simulink model "System_Model_Updated_2"  (R2021a)
settings: Solver=VariableStepAuto  StartTime=0.0  StopTime=50  RelTol=1e-3
libraries: pid_lib x4, vrlib x1, sharedutil x1, sharedtransform x1
settings Model: Creator=Hameed  LastModifiedBy=Hameed

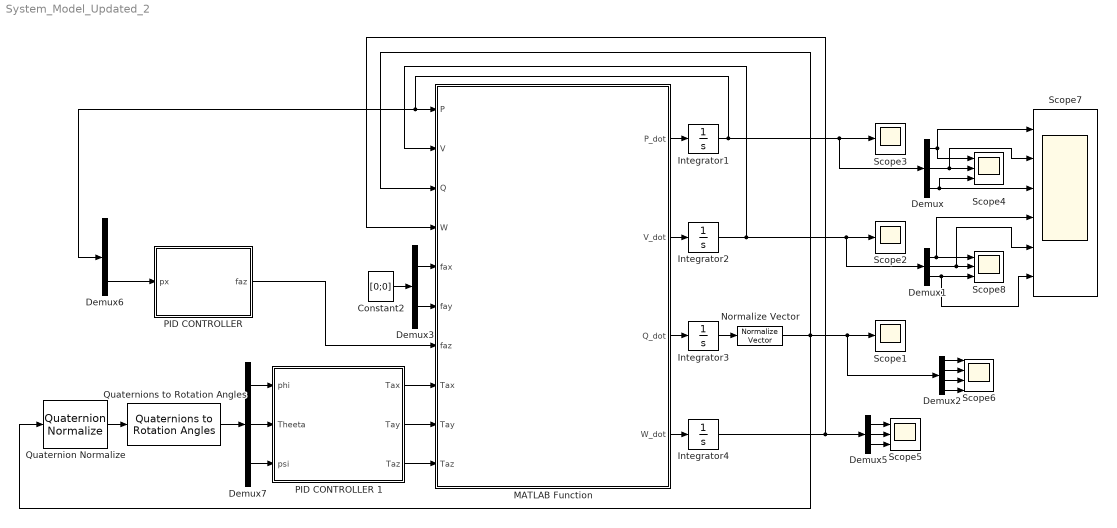
== system System_Model_Updated_2 ==
  Constant2 : Constant  Value=[0;0]  VectorParams1D=off
  Demux{,1,5..7} (5 alike) : Demux  Outputs=3
  Demux2 : Demux
  Demux3 : Demux  Outputs=2
  Integrator1 : Integrator  InitialCondition=[0;0;0]
  Integrator2 : Integrator  InitialCondition=[0;0;0]
  Integrator3 : Integrator  InitialCondition=[1;0;0;0]
  Integrator4 : Integrator  InitialCondition=[0;0;0]
  MATLAB Function : MATLAB Function  TreatAsAtomicUnit=on
  Normalize Vector : vrlib/Utilities/Normalize Vector  maxzero=0
  "PID CONTROLLER " : Subsystem
  PID CONTROLLER 1 : Subsystem
  Quaternion Normalize : sharedutil/Quaternion Normalize  aMode=aMode
      settings: SourceProductBaseCode=AE,PW,DR,MT,UV,VE
  Quaternions to Rotation Angles : sharedtransform/Quaternions to Rotation Angles  rotationOrder=ZYX  aMode=aMode
      settings: SourceProductBaseCode=AE,PW,DR,MT,UV,VE
  Scope1 : Scope
  Scope2 : Scope
  Scope3 : Scope
  Scope4 : Scope  NumInputPorts=3
  Scope5 : Scope  NumInputPorts=3
  Scope6 : Scope  NumInputPorts=4
  Scope7 : Scope  NumInputPorts=6
  Scope8 : Scope  NumInputPorts=3
  wires:
  Demux2/2 -> Scope6/2
  PID CONTROLLER 1/3(Taz) -> MATLAB Function/10(Taz)
  Demux/1 -> Scope4/1, Scope7/1
  Integrator4/1 -> Demux5/1, MATLAB Function/4(W)
  Demux6/3 -> "PID CONTROLLER "/1(px)
  MATLAB Function/2(V_dot) -> Integrator2/1
  Demux7/2 -> PID CONTROLLER 1/2(Theeta)
  PID CONTROLLER 1/1(Tax) -> MATLAB Function/8(Tax)
  Integrator1/1 -> Scope3/1, Demux/1, MATLAB Function/1(P), Demux6/1
  Demux1/3 -> Scope8/3, Scope7/6
  MATLAB Function/4(W_dot) -> Integrator4/1
  Integrator2/1 -> Demux1/1, Scope2/1, MATLAB Function/2(V)
  Integrator3/1 -> Normalize Vector/1
  Quaternion Normalize/1 -> Quaternions to Rotation Angles/1
  Demux/2 -> Scope4/2, Scope7/2
  Demux3/2 -> MATLAB Function/6(fay)
  PID CONTROLLER 1/2(Tay) -> MATLAB Function/9(Tay)
  Demux7/1 -> PID CONTROLLER 1/1(phi)
  Demux3/1 -> MATLAB Function/5(fax)
  MATLAB Function/1(P_dot) -> Integrator1/1
  "PID CONTROLLER "/1(faz) -> MATLAB Function/7(faz)
  Demux2/1 -> Scope6/1
  Demux5/2 -> Scope5/2
  Normalize Vector/1 -> Quaternion Normalize/1, Scope1/1, Demux2/1, MATLAB Function/3(Q)
  Demux/3 -> Scope4/3, Scope7/3
  Demux7/3 -> PID CONTROLLER 1/3(psi)
  Demux2/4 -> Scope6/4
  Demux1/1 -> Scope8/1, Scope7/4
  Quaternions to Rotation Angles/1 -> Demux7/1
  Demux1/2 -> Scope7/5, Scope8/2
  Demux5/1 -> Scope5/1
  Demux2/3 -> Scope6/3
  MATLAB Function/3(Q_dot) -> Integrator3/1
  Demux5/3 -> Scope5/3
  Constant2/1 -> Demux3/1

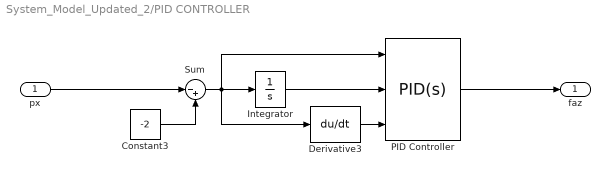
== system System_Model_Updated_2/PID CONTROLLER  ==
  px : Inport
  Constant3 : Constant  Value=-2  VectorParams1D=off
  Derivative3 : Derivative
  Integrator : Integrator
  PID Controller : pid_lib/PID Controller  Controller=PID  Form=Parallel  TimeDomain=Continuous-time  UseExternalTs=off  SampleTime=-1  IntegratorMethod=Forward Euler  FilterMethod=Forward Euler  ControllerParametersSource=internal  P=50  I=60  D=30  UseFilter=on  N=100  TunerSelectOption=Transfer Function Based (PID Tuner App)  InitialConditionSource=external  InitialConditionForIntegrator=0  InitialConditionForFilter=0  DifferentiatorICPrevScaledInput=0  ExternalReset=none  TrackingMode=off  Kt=1  LimitOutput=off  SatLimitsSource=internal  UpperSaturationLimit=inf  LowerSaturationLimit=-inf  LinearizeAsGain=on  AntiWindupMode=none  Kb=1  POutMin=[]  POutMax=[]  IOutMin=[]  IOutMax=[]  DOutMin=[]  DOutMax=[]  NOutMin=[]  NOutMax=[]  SumOutMin=[]  SumOutMax=[]  SaturationOutMin=[]  SaturationOutMax=[]  PParamMin=[]  PParamMax=[]  IParamMin=[]  IParamMax=[]  DParamMin=[]  DParamMax=[]  NParamMin=[]  NParamMax=[]  KbParamMin=[]  KbParamMax=[]  KtParamMin=[]  KtParamMax=[]  KbOutMin=[]  KbOutMax=[]  KtOutMin=[]  KtOutMax=[]  IntegratorOutMin=[]  IntegratorOutMax=[]  FilterOutMin=[]  FilterOutMax=[]  SumI1OutMin=[]  SumI1OutMax=[]  SumI2OutMin=[]  SumI2OutMax=[]  SumI3OutMin=[]  SumI3OutMax=[]  SumI4OutMin=[]  SumI4OutMax=[]  SumDOutMin=[]  SumDOutMax=[]  DifferentiatorOutMin=[]  DifferentiatorOutMax=[]  FilterDiffOutCoefMin=[]  FilterDiffOutCoefMax=[]  ReciprocalOutMin=[]  ReciprocalOutMax=[]  SumDenOutMin=[]  SumDenOutMax=[]  SumNumOutMin=[]  SumNumOutMax=[]  DivideOutMin=[]  DivideOutMax=[]  UdiffTsProdOutMin=[]  UdiffTsProdOutMax=[]  NTsProdOutMin=[]  NTsProdOutMax=[]  UintegralTsProdOutMin=[]  UintegralTsProdOutMax=[]  UngainTsProdOutMin=[]  UngainTsProdOutMax=[]  IntegratorContinuousStateAttributes=''  IntegratorStateMustResolveToSignalObject=off  IntegratorRTWStateStorageClass=Auto  FilterContinuousStateAttributes=''  FilterStateMustResolveToSignalObject=off  FilterRTWStateStorageClass=Auto  ParallelPVariant=InternalParameters  IdealPVariant=Disabled  IVariant=InternalParameters  DVariant=InternalParameters  IntegratorVariant=Continuous  SatVariant=Disabled  AWVariant=Passthrough  PCopyVariant=Disabled  TRVariant=Disabled  FdbkBlocksVariant=Forward  IdealPFdbkVariant=Disabled  SatFdbkVariant=Disabled  DerivativeFilterVariant=ContFilter  NVariant=InternalParameters  NCopyVariant=Disabled  FilterICVariant=ExternalICs  IntegratorICVariant=ExternalICs  ExternalResetVariant=Disabled  TRSumVariant=Passthrough  SumFdbkVariant=Disabled  SumVariant=Sum_PID  TsampFilterVariant=InternalTs  TsampNgainVariant=Passthrough  TsampIntegralVariant=Passthrough  ExternalSaturationOutDataTypeStr=Inherit: Same as second input
  Sum : Sum  Inputs=|-+
  faz : Outport
  wires:
  Derivative3/1 -> PID Controller/3
  px/1 -> Sum/1
  Constant3/1 -> Sum/2
  Integrator/1 -> PID Controller/2
  Sum/1 -> Derivative3/1, PID Controller/1, Integrator/1
  PID Controller/1 -> faz/1

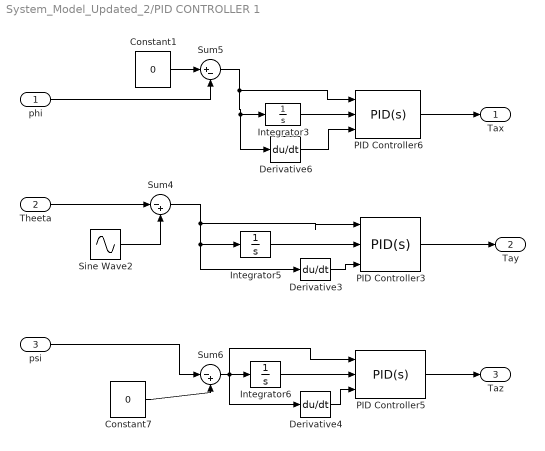
== system System_Model_Updated_2/PID CONTROLLER 1 ==
  phi : Inport
  Theeta : Inport  Port=2
  psi : Inport  Port=3
  Constant1 : Constant  Value=0  VectorParams1D=off
  Constant7 : Constant  Value=0  VectorParams1D=off
  Derivative3 : Derivative
  Derivative4 : Derivative
  Derivative6 : Derivative
  Integrator3 : Integrator
  Integrator5 : Integrator
  Integrator6 : Integrator
  PID Controller3 : pid_lib/PID Controller  Controller=PID  Form=Parallel  TimeDomain=Continuous-time  UseExternalTs=off  SampleTime=-1  IntegratorMethod=Forward Euler  FilterMethod=Forward Euler  ControllerParametersSource=internal  P=20  I=1  D=10  UseFilter=on  N=100  TunerSelectOption=Transfer Function Based (PID Tuner App)  InitialConditionSource=external  InitialConditionForIntegrator=0  InitialConditionForFilter=0  DifferentiatorICPrevScaledInput=0  ExternalReset=none  TrackingMode=off  Kt=1  LimitOutput=off  SatLimitsSource=internal  UpperSaturationLimit=inf  LowerSaturationLimit=-inf  LinearizeAsGain=on  AntiWindupMode=none  Kb=1  POutMin=[]  POutMax=[]  IOutMin=[]  IOutMax=[]  DOutMin=[]  DOutMax=[]  NOutMin=[]  NOutMax=[]  SumOutMin=[]  SumOutMax=[]  SaturationOutMin=[]  SaturationOutMax=[]  PParamMin=[]  PParamMax=[]  IParamMin=[]  IParamMax=[]  DParamMin=[]  DParamMax=[]  NParamMin=[]  NParamMax=[]  KbParamMin=[]  KbParamMax=[]  KtParamMin=[]  KtParamMax=[]  KbOutMin=[]  KbOutMax=[]  KtOutMin=[]  KtOutMax=[]  IntegratorOutMin=[]  IntegratorOutMax=[]  FilterOutMin=[]  FilterOutMax=[]  SumI1OutMin=[]  SumI1OutMax=[]  SumI2OutMin=[]  SumI2OutMax=[]  SumI3OutMin=[]  SumI3OutMax=[]  SumI4OutMin=[]  SumI4OutMax=[]  SumDOutMin=[]  SumDOutMax=[]  DifferentiatorOutMin=[]  DifferentiatorOutMax=[]  FilterDiffOutCoefMin=[]  FilterDiffOutCoefMax=[]  ReciprocalOutMin=[]  ReciprocalOutMax=[]  SumDenOutMin=[]  SumDenOutMax=[]  SumNumOutMin=[]  SumNumOutMax=[]  DivideOutMin=[]  DivideOutMax=[]  UdiffTsProdOutMin=[]  UdiffTsProdOutMax=[]  NTsProdOutMin=[]  NTsProdOutMax=[]  UintegralTsProdOutMin=[]  UintegralTsProdOutMax=[]  UngainTsProdOutMin=[]  UngainTsProdOutMax=[]  IntegratorContinuousStateAttributes=''  IntegratorStateMustResolveToSignalObject=off  IntegratorRTWStateStorageClass=Auto  FilterContinuousStateAttributes=''  FilterStateMustResolveToSignalObject=off  FilterRTWStateStorageClass=Auto  ParallelPVariant=InternalParameters  IdealPVariant=Disabled  IVariant=InternalParameters  DVariant=InternalParameters  IntegratorVariant=Continuous  SatVariant=Disabled  AWVariant=Passthrough  PCopyVariant=Disabled  TRVariant=Disabled  FdbkBlocksVariant=Forward  IdealPFdbkVariant=Disabled  SatFdbkVariant=Disabled  DerivativeFilterVariant=ContFilter  NVariant=InternalParameters  NCopyVariant=Disabled  FilterICVariant=ExternalICs  IntegratorICVariant=ExternalICs  ExternalResetVariant=Disabled  TRSumVariant=Passthrough  SumFdbkVariant=Disabled  SumVariant=Sum_PID  TsampFilterVariant=InternalTs  TsampNgainVariant=Passthrough  TsampIntegralVariant=Passthrough  ExternalSaturationOutDataTypeStr=Inherit: Same as second input
  PID Controller5 : pid_lib/PID Controller  Controller=PID  Form=Parallel  TimeDomain=Continuous-time  UseExternalTs=off  SampleTime=-1  IntegratorMethod=Forward Euler  FilterMethod=Forward Euler  ControllerParametersSource=internal  P=20  I=1  D=10  UseFilter=on  N=100  TunerSelectOption=Transfer Function Based (PID Tuner App)  InitialConditionSource=external  InitialConditionForIntegrator=0  InitialConditionForFilter=0  DifferentiatorICPrevScaledInput=0  ExternalReset=none  TrackingMode=off  Kt=1  LimitOutput=off  SatLimitsSource=internal  UpperSaturationLimit=inf  LowerSaturationLimit=-inf  LinearizeAsGain=on  AntiWindupMode=none  Kb=1  POutMin=[]  POutMax=[]  IOutMin=[]  IOutMax=[]  DOutMin=[]  DOutMax=[]  NOutMin=[]  NOutMax=[]  SumOutMin=[]  SumOutMax=[]  SaturationOutMin=[]  SaturationOutMax=[]  PParamMin=[]  PParamMax=[]  IParamMin=[]  IParamMax=[]  DParamMin=[]  DParamMax=[]  NParamMin=[]  NParamMax=[]  KbParamMin=[]  KbParamMax=[]  KtParamMin=[]  KtParamMax=[]  KbOutMin=[]  KbOutMax=[]  KtOutMin=[]  KtOutMax=[]  IntegratorOutMin=[]  IntegratorOutMax=[]  FilterOutMin=[]  FilterOutMax=[]  SumI1OutMin=[]  SumI1OutMax=[]  SumI2OutMin=[]  SumI2OutMax=[]  SumI3OutMin=[]  SumI3OutMax=[]  SumI4OutMin=[]  SumI4OutMax=[]  SumDOutMin=[]  SumDOutMax=[]  DifferentiatorOutMin=[]  DifferentiatorOutMax=[]  FilterDiffOutCoefMin=[]  FilterDiffOutCoefMax=[]  ReciprocalOutMin=[]  ReciprocalOutMax=[]  SumDenOutMin=[]  SumDenOutMax=[]  SumNumOutMin=[]  SumNumOutMax=[]  DivideOutMin=[]  DivideOutMax=[]  UdiffTsProdOutMin=[]  UdiffTsProdOutMax=[]  NTsProdOutMin=[]  NTsProdOutMax=[]  UintegralTsProdOutMin=[]  UintegralTsProdOutMax=[]  UngainTsProdOutMin=[]  UngainTsProdOutMax=[]  IntegratorContinuousStateAttributes=''  IntegratorStateMustResolveToSignalObject=off  IntegratorRTWStateStorageClass=Auto  FilterContinuousStateAttributes=''  FilterStateMustResolveToSignalObject=off  FilterRTWStateStorageClass=Auto  ParallelPVariant=InternalParameters  IdealPVariant=Disabled  IVariant=InternalParameters  DVariant=InternalParameters  IntegratorVariant=Continuous  SatVariant=Disabled  AWVariant=Passthrough  PCopyVariant=Disabled  TRVariant=Disabled  FdbkBlocksVariant=Forward  IdealPFdbkVariant=Disabled  SatFdbkVariant=Disabled  DerivativeFilterVariant=ContFilter  NVariant=InternalParameters  NCopyVariant=Disabled  FilterICVariant=ExternalICs  IntegratorICVariant=ExternalICs  ExternalResetVariant=Disabled  TRSumVariant=Passthrough  SumFdbkVariant=Disabled  SumVariant=Sum_PID  TsampFilterVariant=InternalTs  TsampNgainVariant=Passthrough  TsampIntegralVariant=Passthrough  ExternalSaturationOutDataTypeStr=Inherit: Same as second input
  PID Controller6 : pid_lib/PID Controller  Controller=PID  Form=Parallel  TimeDomain=Continuous-time  UseExternalTs=off  SampleTime=-1  IntegratorMethod=Forward Euler  FilterMethod=Forward Euler  ControllerParametersSource=internal  P=20  I=1  D=10  UseFilter=on  N=100  TunerSelectOption=Transfer Function Based (PID Tuner App)  InitialConditionSource=external  InitialConditionForIntegrator=0  InitialConditionForFilter=0  DifferentiatorICPrevScaledInput=0  ExternalReset=none  TrackingMode=off  Kt=1  LimitOutput=off  SatLimitsSource=internal  UpperSaturationLimit=inf  LowerSaturationLimit=-inf  LinearizeAsGain=on  AntiWindupMode=none  Kb=1  POutMin=[]  POutMax=[]  IOutMin=[]  IOutMax=[]  DOutMin=[]  DOutMax=[]  NOutMin=[]  NOutMax=[]  SumOutMin=[]  SumOutMax=[]  SaturationOutMin=[]  SaturationOutMax=[]  PParamMin=[]  PParamMax=[]  IParamMin=[]  IParamMax=[]  DParamMin=[]  DParamMax=[]  NParamMin=[]  NParamMax=[]  KbParamMin=[]  KbParamMax=[]  KtParamMin=[]  KtParamMax=[]  KbOutMin=[]  KbOutMax=[]  KtOutMin=[]  KtOutMax=[]  IntegratorOutMin=[]  IntegratorOutMax=[]  FilterOutMin=[]  FilterOutMax=[]  SumI1OutMin=[]  SumI1OutMax=[]  SumI2OutMin=[]  SumI2OutMax=[]  SumI3OutMin=[]  SumI3OutMax=[]  SumI4OutMin=[]  SumI4OutMax=[]  SumDOutMin=[]  SumDOutMax=[]  DifferentiatorOutMin=[]  DifferentiatorOutMax=[]  FilterDiffOutCoefMin=[]  FilterDiffOutCoefMax=[]  ReciprocalOutMin=[]  ReciprocalOutMax=[]  SumDenOutMin=[]  SumDenOutMax=[]  SumNumOutMin=[]  SumNumOutMax=[]  DivideOutMin=[]  DivideOutMax=[]  UdiffTsProdOutMin=[]  UdiffTsProdOutMax=[]  NTsProdOutMin=[]  NTsProdOutMax=[]  UintegralTsProdOutMin=[]  UintegralTsProdOutMax=[]  UngainTsProdOutMin=[]  UngainTsProdOutMax=[]  IntegratorContinuousStateAttributes=''  IntegratorStateMustResolveToSignalObject=off  IntegratorRTWStateStorageClass=Auto  FilterContinuousStateAttributes=''  FilterStateMustResolveToSignalObject=off  FilterRTWStateStorageClass=Auto  ParallelPVariant=InternalParameters  IdealPVariant=Disabled  IVariant=InternalParameters  DVariant=InternalParameters  IntegratorVariant=Continuous  SatVariant=Disabled  AWVariant=Passthrough  PCopyVariant=Disabled  TRVariant=Disabled  FdbkBlocksVariant=Forward  IdealPFdbkVariant=Disabled  SatFdbkVariant=Disabled  DerivativeFilterVariant=ContFilter  NVariant=InternalParameters  NCopyVariant=Disabled  FilterICVariant=ExternalICs  IntegratorICVariant=ExternalICs  ExternalResetVariant=Disabled  TRSumVariant=Passthrough  SumFdbkVariant=Disabled  SumVariant=Sum_PID  TsampFilterVariant=InternalTs  TsampNgainVariant=Passthrough  TsampIntegralVariant=Passthrough  ExternalSaturationOutDataTypeStr=Inherit: Same as second input
  Sine Wave2 : Sin  Amplitude=0.1  Frequency=2*pi*0.1  SampleTime=0
  Sum4 : Sum  Inputs=|-+
  Sum5 : Sum  Inputs=|+-
  Sum6 : Sum  Inputs=|-+
  Tax : Outport
  Tay : Outport  Port=2
  Taz : Outport  Port=3
  wires:
  Derivative6/1 -> PID Controller6/3
  PID Controller5/1 -> Taz/1
  PID Controller3/1 -> Tay/1
  Sum4/1 -> Derivative3/1, Integrator5/1, PID Controller3/1
  Derivative4/1 -> PID Controller5/3
  Integrator6/1 -> PID Controller5/2
  Constant7/1 -> Sum6/2
  Integrator5/1 -> PID Controller3/2
  Derivative3/1 -> PID Controller3/3
  psi/1 -> Sum6/1
  Sine Wave2/1 -> Sum4/2
  phi/1 -> Sum5/2
  PID Controller6/1 -> Tax/1
  Sum6/1 -> Derivative4/1, Integrator6/1, PID Controller5/1
  Integrator3/1 -> PID Controller6/2
  Sum5/1 -> Derivative6/1, Integrator3/1, PID Controller6/1
  Constant1/1 -> Sum5/1
  Theeta/1 -> Sum4/1

== matlab function System_Model_Updated_2/MATLAB Function ==
  data: P input; P_dot output; V input; Q input; W input; V_dot output; Q_dot output; W_dot output; fax input; fay input; faz input; Tax input; Tay input; Taz input
function [P_dot,V_dot,Q_dot,W_dot]= fcn(P,V,Q,W,fax,fay,faz,Tax,Tay,Taz)
clc
m=5;

%%% phi=Q(2); % theta=Q(3); % psi=Q(4);

% Rz=[cos(psi) sin(psi) 0;-sin(psi)) cos(psi) 0;0 0 1];
% Rx=[1 0 0;0 cos(phi) sin(phi);0 -sin(phi) cos(phi)];
% Ry=[cos(theta) 0 -sin(theta);0 1 0;sin(theta) 0 cos(theta)];

Rz=[cos(Q(4)) sin(Q(4)) 0; -sin(Q(4)) cos(Q(4)) 0; 0 0 1];
Rx=[1 0 0; 0 cos(Q(2)) sin(Q(2)); 0 -sin(Q(2)) cos(Q(2))];
Ry=[cos(Q(3)) 0 -sin(Q(3)); 0 1 0; sin(Q(3)) 0 cos(Q(3))];

Rb=Rz*Ry*Rx;
Rs=[1 0 0;
    0 0 -1;
    0 1 0 ];

%Rs=[1 0 0;0 -1 0;0 0 -1];
%lambda=L;
L=0;
%L=1;
Rd=[1 0 0;
    0 1 0;
    0 0 1-L];

SL=Rs*Rd*transpose(Rs);

rT=[0.5;0;0];

Ixx=1;
Iyy=1;
Izz=1;
J=[Ixx 0 0;0 Iyy 0;0 0 Izz];

g=9.8;
dF=[0;0;0];
fc=[0;0;0];
rcom=[0;0;0];
dT=[0;0;0];

fa=[fax;fay;faz];
ta=[Tax;Tay;Taz];

ab=(m^-1)*((Rb*fa)+(L*fc)+dF)+[0;0;g];

% T=[0 -sin(Q(2)) cos(Q(2))*sin(Q(3));
% 0 cos(Q(2)) sin(Q(2))*sin(Q(3));
% 1 0 cos(Q(3))];

Sq=[0 -Q(4) Q(3);
    Q(4) 0 -Q(2);
    -Q(3) Q(2) 0];

eata_dot=[Q(2);Q(3);Q(4)]
%w=T*eata_dot;

h=J*W;
h1=transpose(Rb)*[0;0;m*g];
h2=L*transpose(Rb)*fc;

P_dot=SL*V;

Qw_dot=-1/2*[Q(2) Q(3) Q(4)]*W;
Qv_dot=1/2*(Q(1)*J-Sq)*W;

% Qw_dot=-1/2*[Q(2) Q(3) Q(4)]*W
% Qv_dot=1/2*(Q(1)*J-Sq)*W;
Q_dot=[Qw_dot;Qv_dot];

W_dot=(inv(J))*(ta-cross(W,h)+cross(rcom,h1)+cross(rT,h2)+dT);

V_dot=SL*((ab)+Rb*(cross(W_dot,rT)+(cross(W,cross(W,rT)))));
